simulink model "Lab6_1"  (R2025a)
settings: Solver=FixedStepDiscrete  StartTime=0.0  StopTime=A.len*16 + 52  FixedStep=1  RelTol=1e-3
PostLoadFcn:
  | A = DEScfg_axi('$0102040810204080', 'This is a default input - make it your own!', 'encrypt')
undefined symbols (not defined in the file): AXI4, Lite, xc7z020clg484
libraries: hdlBasic x260, vmcUtilities x1
(part 2 of 2)

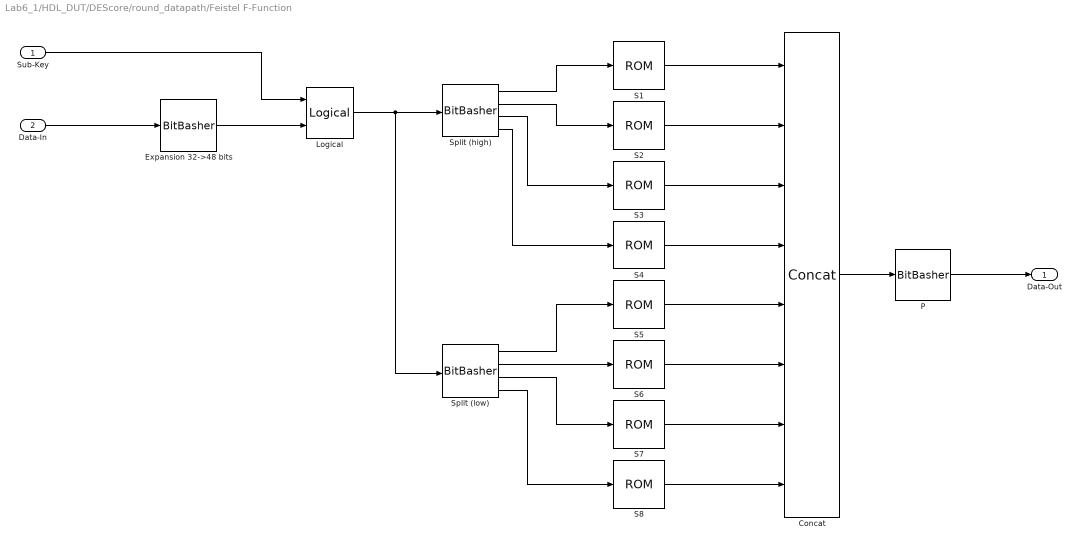
== system Lab6_1/HDL_DUT/DEScore/round_datapath/Feistel F-Function ==
  Sub-Key : Inport
  Data-In : Inport  Port=2
  Concat : hdlBasic/Concat  num_inputs=8  XmcBlockStatus=1  maskContainerNames=group1  block_type=concat  block_config=sysgen:Concat_config
  Expansion 32->48 bits : hdlBasic/BitBasher  bitexpr=x={a[0],a[31:27],a[28:23],a[24:19],a[20:15],a[16:11],a[12:7],a[8:3],a[4:0],a[31]}  display_expr=off  sr_1=x  arith_type1=Unsigned  bin_pt1=0  sr_2=y  arith_type2=Unsigned  bin_pt2=0  sr_3=z  arith_type3=Unsigned  bin_pt3=0  sr_4=t  arith_type4=Unsigned  bin_pt4=0  XmcBlockStatus=1  maskContainerNames=group1  block_type=bitbasher  block_config=sysgen:BitBasher_config
  Logical : hdlBasic/Logical  logical_function=XOR  inputs=2  en=off  latency=0  precision=Full  arith_type=Unsigned  n_bits=16  bin_pt=0  align_bp=on  overflow=[]  quantization=[]  XmcBlockStatus=1  maskContainerNames=tabcontainer1  block_type=logical  block_config=sysgen:Logical_config
  P : hdlBasic/BitBasher  bitexpr=out={a[16], a[25], a[12], a[11], a[3], a[20], a[4], a[15], a[31], a[17], a[9], a[6], a[27], a[14], a[1], a[22], a[30], a[24], a[8], a[18], a[0], a[5], a[29], a[23], a[13], a[19], a[2], a[26], a[10], a[21], a[28], a[7]}  display_expr=off  sr_1=out  arith_type1=Unsigned  bin_pt1=0  sr_2=2  arith_type2=Unsigned  bin_pt2=0  sr_3=3  arith_type3=Unsigned  bin_pt3=0  sr_4=4  arith_type4=Unsigned  bin_pt4=0  XmcBlockStatus=1  maskContainerNames=group1  block_type=bitbasher  block_config=sysgen:BitBasher_config
  S1 : hdlBasic/ROM  depth=64  initVector=[14 0 4 15 13 7 1 4 2 14 15 2 11 13 8 1 3 10 10 6 6 12 12 11 5 9 9 5 0 3 7 8 4 15 1 12 14 8 8 2 13 4 6 9 2 1 11 7 15 5 12 11 9 3 7 14 3 10 10 0 5 6 0 13]  distributed_mem=Distributed memory  rst=off  init_reg=0  en=off  latency=0  gui_display_data_type=Fixed-point  arith_type=Unsigned  n_bits=4  bin_pt=0  preci_type=Single  exp_width=8  frac_width=24  optimize=Area  use_rpm=on  simulation_type=fast_sim  XmcBlockStatus=1  maskContainerNames=tabcontainer1  block_type=sprom  block_config=sysgen:SPROM_config
  S2 : hdlBasic/ROM  depth=64  initVector=[15 3 1 13 8 4 14 7 6 15 11 2 3 8 4 14 9 12 7 0 2 1 13 10 12 6 0 9 5 11 10 5 0 13 14 8 7 10 11 1 10 3 4 15 13 4 1 2 5 11 8 6 12 7 6 12 9 0 3 5 2 14 15 9]  distributed_mem=Distributed memory  rst=off  init_reg=0  en=off  latency=0  gui_display_data_type=Fixed-point  arith_type=Unsigned  n_bits=4  bin_pt=0  preci_type=Single  exp_width=8  frac_width=24  optimize=Area  use_rpm=on  simulation_type=fast_sim  XmcBlockStatus=1  maskContainerNames=tabcontainer1  block_type=sprom  block_config=sysgen:SPROM_config
  S3 : hdlBasic/ROM  depth=64  initVector=[10 13 0 7 9 0 14 9 6 3 3 4 15 6 5 10 1 2 13 8 12 5 7 14 11 12 4 11 2 15 8 1 13 1 6 10 4 13 9 0 8 6 15 9 3 8 0 7 11 4 1 15 2 14 12 3 5 11 10 5 14 2 7 12]  distributed_mem=Distributed memory  rst=off  init_reg=0  en=off  latency=0  gui_display_data_type=Fixed-point  arith_type=Unsigned  n_bits=4  bin_pt=0  preci_type=Single  exp_width=8  frac_width=24  optimize=Area  use_rpm=on  simulation_type=fast_sim  XmcBlockStatus=1  maskContainerNames=tabcontainer1  block_type=sprom  block_config=sysgen:SPROM_config
  S4 : hdlBasic/ROM  depth=64  initVector=[7 13 13 8 14 11 3 5 0 6 6 15 9 0 10 3 1 4 2 7 8 2 5 12 11 1 12 10 4 14 15 9 10 3 6 15 9 0 0 6 12 10 11 1 7 13 13 8 15 9 1 4 3 5 14 11 5 12 2 7 8 2 4 14]  distributed_mem=Distributed memory  rst=off  init_reg=0  en=off  latency=0  gui_display_data_type=Fixed-point  arith_type=Unsigned  n_bits=4  bin_pt=0  preci_type=Single  exp_width=8  frac_width=24  optimize=Area  use_rpm=on  simulation_type=fast_sim  XmcBlockStatus=1  maskContainerNames=tabcontainer1  block_type=sprom  block_config=sysgen:SPROM_config
  S5 : hdlBasic/ROM  depth=64  initVector=[2 14 12 11 4 2 1 12 7 4 10 7 11 13 6 1 8 5 5 0 3 15 15 10 13 3 0 9 14 8 9 6 4 11 2 8 1 12 11 7 10 1 13 14 7 2 8 13 15 6 9 15 12 0 5 9 6 10 3 4 0 5 14 3]  distributed_mem=Distributed memory  rst=off  init_reg=0  en=off  latency=0  gui_display_data_type=Fixed-point  arith_type=Unsigned  n_bits=4  bin_pt=0  preci_type=Single  exp_width=8  frac_width=24  optimize=Area  use_rpm=on  simulation_type=fast_sim  XmcBlockStatus=1  maskContainerNames=tabcontainer1  block_type=sprom  block_config=sysgen:SPROM_config
  S6 : hdlBasic/ROM  depth=64  initVector=[12 10 1 15 10 4 15 2 9 7 2 12 6 9 8 5 0 6 13 1 3 13 4 14 14 0 7 11 5 3 11 8 9 4 14 3 15 2 5 12 2 9 8 5 12 15 3 10 7 11 0 14 4 1 10 7 1 6 13 0 11 8 6 13]  distributed_mem=Distributed memory  rst=off  init_reg=0  en=off  latency=0  gui_display_data_type=Fixed-point  arith_type=Unsigned  n_bits=4  bin_pt=0  preci_type=Single  exp_width=8  frac_width=24  optimize=Area  use_rpm=on  simulation_type=fast_sim  XmcBlockStatus=1  maskContainerNames=tabcontainer1  block_type=sprom  block_config=sysgen:SPROM_config
  S7 : hdlBasic/ROM  depth=64  initVector=[4 13 11 0 2 11 14 7 15 4 0 9 8 1 13 10 3 14 12 3 9 5 7 12 5 2 10 15 6 8 1 6 1 6 4 11 11 13 13 8 12 1 3 4 7 10 14 7 10 9 15 5 6 0 8 15 0 14 5 2 9 3 2 12]  distributed_mem=Distributed memory  rst=off  init_reg=0  en=off  latency=0  gui_display_data_type=Fixed-point  arith_type=Unsigned  n_bits=4  bin_pt=0  preci_type=Single  exp_width=8  frac_width=24  optimize=Area  use_rpm=on  simulation_type=fast_sim  XmcBlockStatus=1  maskContainerNames=tabcontainer1  block_type=sprom  block_config=sysgen:SPROM_config
  S8 : hdlBasic/ROM  depth=64  initVector=[13 1 2 15 8 13 4 8 6 10 15 3 11 7 1 4 10 12 9 5 3 6 14 11 5 0 0 14 12 9 7 2 7 2 11 1 4 14 1 7 9 4 12 10 14 8 2 13 0 15 6 12 10 9 13 0 15 3 3 5 5 6 8 11]  distributed_mem=Distributed memory  rst=off  init_reg=0  en=off  latency=0  gui_display_data_type=Fixed-point  arith_type=Unsigned  n_bits=4  bin_pt=0  preci_type=Single  exp_width=8  frac_width=24  optimize=Area  use_rpm=on  simulation_type=fast_sim  XmcBlockStatus=1  maskContainerNames=tabcontainer1  block_type=sprom  block_config=sysgen:SPROM_config
  Split (high) : hdlBasic/BitBasher  bitexpr=|  display_expr=off  sr_1=a  arith_type1=Unsigned  bin_pt1=0  sr_2=b  arith_type2=Unsigned  bin_pt2=0  sr_3=c  arith_type3=Unsigned  bin_pt3=0  sr_4=d  arith_type4=Unsigned  bin_pt4=0  XmcBlockStatus=1  maskContainerNames=group1  block_type=bitbasher  block_config=sysgen:BitBasher_config
      | a={x[47:42]}
      | b={x[41:36]}
      | c={x[35:30]}
      | d={x[29:24]}
  Split (low) : hdlBasic/BitBasher  bitexpr=|  display_expr=off  sr_1=a  arith_type1=Unsigned  bin_pt1=0  sr_2=b  arith_type2=Unsigned  bin_pt2=0  sr_3=c  arith_type3=Unsigned  bin_pt3=0  sr_4=d  arith_type4=Unsigned  bin_pt4=0  XmcBlockStatus=1  maskContainerNames=group1  block_type=bitbasher  block_config=sysgen:BitBasher_config
      | a={x[23:18]}
      | b={x[17:12]}
      | c={x[11:6]}
      | d={x[5:0]}
  Data-Out : Outport
  wires:
  Split (low)/2 -> S6/1
  Split (low)/3 -> S7/1
  Concat/1 -> P/1
  S4/1 -> Concat/4
  Split (low)/1 -> S5/1
  Split (high)/3 -> S3/1
  S6/1 -> Concat/6
  Split (high)/4 -> S4/1
  S8/1 -> Concat/8
  Data-In/1 -> Expansion 32->48 bits/1
  S1/1 -> Concat/1
  Logical/1 -> Split (low)/1, Split (high)/1
  Sub-Key/1 -> Logical/1
  Expansion 32->48 bits/1 -> Logical/2
  Split (low)/4 -> S8/1
  Split (high)/1 -> S1/1
  Split (high)/2 -> S2/1
  S7/1 -> Concat/7
  S5/1 -> Concat/5
  S2/1 -> Concat/2
  S3/1 -> Concat/3
  P/1 -> Data-Out/1

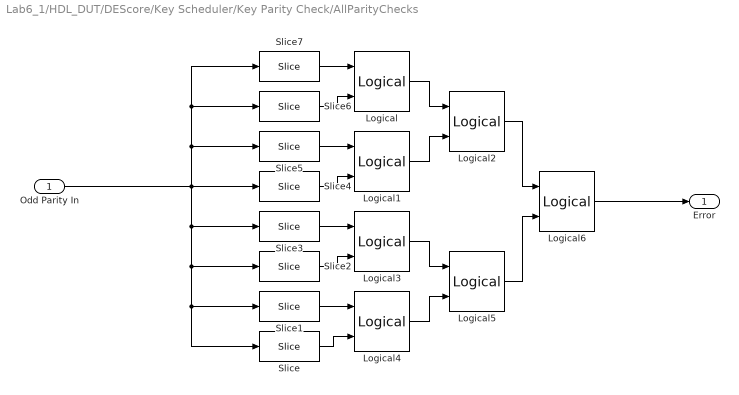
== system Lab6_1/HDL_DUT/DEScore/Key Scheduler/Key Parity Check/AllParityChecks ==
  Odd Parity In : Inport
  Logical{,1..5} (6 alike) : hdlBasic/Logical  logical_function=AND  inputs=2  en=off  latency=0  precision=Full  arith_type=Unsigned  n_bits=16  bin_pt=0  align_bp=on  overflow=[]  quantization=[]  XmcBlockStatus=1  maskContainerNames=tabcontainer1  block_type=logical  block_config=sysgen:Logical_config
  Logical6 : hdlBasic/Logical  logical_function=NAND  inputs=2  en=off  latency=0  precision=Full  arith_type=Unsigned  n_bits=16  bin_pt=0  align_bp=on  overflow=[]  quantization=[]  XmcBlockStatus=1  maskContainerNames=tabcontainer1  block_type=logical  block_config=sysgen:Logical_config
  Slice : hdlBasic/Slice  nbits=1  boolean_output=on  mode=Upper Bit Location + Width  bit1=0  base1=LSB of Input  bit0=0  base0=LSB of Input  XmcBlockStatus=1  maskContainerNames=group1  block_type=slice  block_config=sysgen:Slice_config
  Slice1 : hdlBasic/Slice  nbits=1  boolean_output=on  mode=Upper Bit Location + Width  bit1=1  base1=LSB of Input  bit0=0  base0=LSB of Input  XmcBlockStatus=1  maskContainerNames=group1  block_type=slice  block_config=sysgen:Slice_config
  Slice2 : hdlBasic/Slice  nbits=1  boolean_output=on  mode=Upper Bit Location + Width  bit1=2  base1=LSB of Input  bit0=0  base0=LSB of Input  XmcBlockStatus=1  maskContainerNames=group1  block_type=slice  block_config=sysgen:Slice_config
  Slice3 : hdlBasic/Slice  nbits=1  boolean_output=on  mode=Upper Bit Location + Width  bit1=3  base1=LSB of Input  bit0=0  base0=LSB of Input  XmcBlockStatus=1  maskContainerNames=group1  block_type=slice  block_config=sysgen:Slice_config
  Slice4 : hdlBasic/Slice  nbits=1  boolean_output=on  mode=Upper Bit Location + Width  bit1=4  base1=LSB of Input  bit0=0  base0=LSB of Input  XmcBlockStatus=1  maskContainerNames=group1  block_type=slice  block_config=sysgen:Slice_config
  Slice5 : hdlBasic/Slice  nbits=1  boolean_output=on  mode=Upper Bit Location + Width  bit1=5  base1=LSB of Input  bit0=0  base0=LSB of Input  XmcBlockStatus=1  maskContainerNames=group1  block_type=slice  block_config=sysgen:Slice_config
  Slice6 : hdlBasic/Slice  nbits=1  boolean_output=on  mode=Upper Bit Location + Width  bit1=6  base1=LSB of Input  bit0=0  base0=LSB of Input  XmcBlockStatus=1  maskContainerNames=group1  block_type=slice  block_config=sysgen:Slice_config
  Slice7 : hdlBasic/Slice  nbits=1  boolean_output=on  mode=Upper Bit Location + Width  bit1=7  base1=LSB of Input  bit0=0  base0=LSB of Input  XmcBlockStatus=1  maskContainerNames=group1  block_type=slice  block_config=sysgen:Slice_config
  Error : Outport
  wires:
  Logical/1 -> Logical2/1
  Slice3/1 -> Logical3/1
  Slice1/1 -> Logical4/1
  Logical2/1 -> Logical6/1
  Logical1/1 -> Logical2/2
  Slice/1 -> Logical4/2
  Slice4/1 -> Logical1/2
  Slice5/1 -> Logical1/1
  Logical4/1 -> Logical5/2
  Logical3/1 -> Logical5/1
  Slice7/1 -> Logical/1
  Slice6/1 -> Logical/2
  Slice2/1 -> Logical3/2
  Logical5/1 -> Logical6/2
  Odd Parity In/1 -> Slice7/1, Slice6/1, Slice5/1, Slice/1, Slice1/1, Slice2/1, Slice3/1, Slice4/1
  Logical6/1 -> Error/1

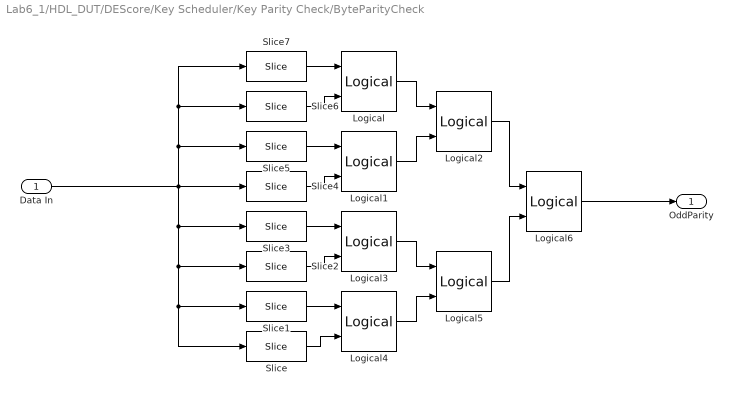
== system Lab6_1/HDL_DUT/DEScore/Key Scheduler/Key Parity Check/ByteParityCheck ==
  Data In : Inport
  Logical{,1..6} (7 alike) : hdlBasic/Logical  logical_function=XOR  inputs=2  en=off  latency=0  precision=Full  arith_type=Unsigned  n_bits=16  bin_pt=0  align_bp=on  overflow=[]  quantization=[]  XmcBlockStatus=1  maskContainerNames=tabcontainer1  block_type=logical  block_config=sysgen:Logical_config
  Slice : hdlBasic/Slice  nbits=1  boolean_output=on  mode=Upper Bit Location + Width  bit1=0  base1=LSB of Input  bit0=0  base0=LSB of Input  XmcBlockStatus=1  maskContainerNames=group1  block_type=slice  block_config=sysgen:Slice_config
  Slice1 : hdlBasic/Slice  nbits=1  boolean_output=on  mode=Upper Bit Location + Width  bit1=1  base1=LSB of Input  bit0=0  base0=LSB of Input  XmcBlockStatus=1  maskContainerNames=group1  block_type=slice  block_config=sysgen:Slice_config
  Slice2 : hdlBasic/Slice  nbits=1  boolean_output=on  mode=Upper Bit Location + Width  bit1=2  base1=LSB of Input  bit0=0  base0=LSB of Input  XmcBlockStatus=1  maskContainerNames=group1  block_type=slice  block_config=sysgen:Slice_config
  Slice3 : hdlBasic/Slice  nbits=1  boolean_output=on  mode=Upper Bit Location + Width  bit1=3  base1=LSB of Input  bit0=0  base0=LSB of Input  XmcBlockStatus=1  maskContainerNames=group1  block_type=slice  block_config=sysgen:Slice_config
  Slice4 : hdlBasic/Slice  nbits=1  boolean_output=on  mode=Upper Bit Location + Width  bit1=4  base1=LSB of Input  bit0=0  base0=LSB of Input  XmcBlockStatus=1  maskContainerNames=group1  block_type=slice  block_config=sysgen:Slice_config
  Slice5 : hdlBasic/Slice  nbits=1  boolean_output=on  mode=Upper Bit Location + Width  bit1=5  base1=LSB of Input  bit0=0  base0=LSB of Input  XmcBlockStatus=1  maskContainerNames=group1  block_type=slice  block_config=sysgen:Slice_config
  Slice6 : hdlBasic/Slice  nbits=1  boolean_output=on  mode=Upper Bit Location + Width  bit1=6  base1=LSB of Input  bit0=0  base0=LSB of Input  XmcBlockStatus=1  maskContainerNames=group1  block_type=slice  block_config=sysgen:Slice_config
  Slice7 : hdlBasic/Slice  nbits=1  boolean_output=on  mode=Upper Bit Location + Width  bit1=7  base1=LSB of Input  bit0=0  base0=LSB of Input  XmcBlockStatus=1  maskContainerNames=group1  block_type=slice  block_config=sysgen:Slice_config
  OddParity : Outport
  wires:
  Logical/1 -> Logical2/1
  Slice3/1 -> Logical3/1
  Slice1/1 -> Logical4/1
  Logical2/1 -> Logical6/1
  Logical1/1 -> Logical2/2
  Slice/1 -> Logical4/2
  Slice4/1 -> Logical1/2
  Slice5/1 -> Logical1/1
  Logical4/1 -> Logical5/2
  Logical3/1 -> Logical5/1
  Slice7/1 -> Logical/1
  Slice6/1 -> Logical/2
  Slice2/1 -> Logical3/2
  Logical5/1 -> Logical6/2
  Data In/1 -> Slice7/1, Slice6/1, Slice5/1, Slice/1, Slice1/1, Slice2/1, Slice3/1, Slice4/1
  Logical6/1 -> OddParity/1

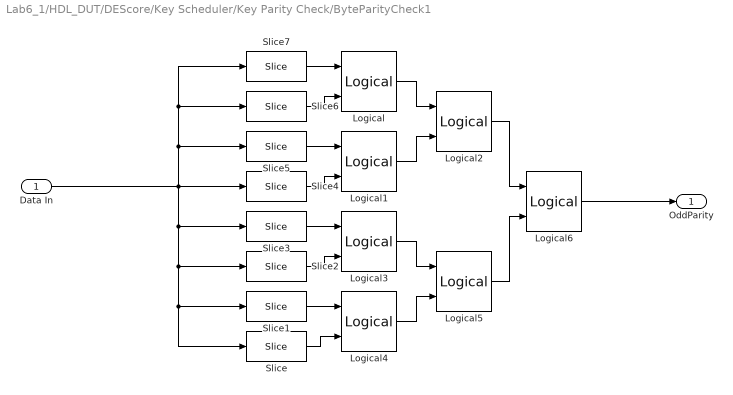
== system Lab6_1/HDL_DUT/DEScore/Key Scheduler/Key Parity Check/ByteParityCheck1 ==
  Data In : Inport
  Logical{,1..6} (7 alike) : hdlBasic/Logical  logical_function=XOR  inputs=2  en=off  latency=0  precision=Full  arith_type=Unsigned  n_bits=16  bin_pt=0  align_bp=on  overflow=[]  quantization=[]  XmcBlockStatus=1  maskContainerNames=tabcontainer1  block_type=logical  block_config=sysgen:Logical_config
  Slice : hdlBasic/Slice  nbits=1  boolean_output=on  mode=Upper Bit Location + Width  bit1=0  base1=LSB of Input  bit0=0  base0=LSB of Input  XmcBlockStatus=1  maskContainerNames=group1  block_type=slice  block_config=sysgen:Slice_config
  Slice1 : hdlBasic/Slice  nbits=1  boolean_output=on  mode=Upper Bit Location + Width  bit1=1  base1=LSB of Input  bit0=0  base0=LSB of Input  XmcBlockStatus=1  maskContainerNames=group1  block_type=slice  block_config=sysgen:Slice_config
  Slice2 : hdlBasic/Slice  nbits=1  boolean_output=on  mode=Upper Bit Location + Width  bit1=2  base1=LSB of Input  bit0=0  base0=LSB of Input  XmcBlockStatus=1  maskContainerNames=group1  block_type=slice  block_config=sysgen:Slice_config
  Slice3 : hdlBasic/Slice  nbits=1  boolean_output=on  mode=Upper Bit Location + Width  bit1=3  base1=LSB of Input  bit0=0  base0=LSB of Input  XmcBlockStatus=1  maskContainerNames=group1  block_type=slice  block_config=sysgen:Slice_config
  Slice4 : hdlBasic/Slice  nbits=1  boolean_output=on  mode=Upper Bit Location + Width  bit1=4  base1=LSB of Input  bit0=0  base0=LSB of Input  XmcBlockStatus=1  maskContainerNames=group1  block_type=slice  block_config=sysgen:Slice_config
  Slice5 : hdlBasic/Slice  nbits=1  boolean_output=on  mode=Upper Bit Location + Width  bit1=5  base1=LSB of Input  bit0=0  base0=LSB of Input  XmcBlockStatus=1  maskContainerNames=group1  block_type=slice  block_config=sysgen:Slice_config
  Slice6 : hdlBasic/Slice  nbits=1  boolean_output=on  mode=Upper Bit Location + Width  bit1=6  base1=LSB of Input  bit0=0  base0=LSB of Input  XmcBlockStatus=1  maskContainerNames=group1  block_type=slice  block_config=sysgen:Slice_config
  Slice7 : hdlBasic/Slice  nbits=1  boolean_output=on  mode=Upper Bit Location + Width  bit1=7  base1=LSB of Input  bit0=0  base0=LSB of Input  XmcBlockStatus=1  maskContainerNames=group1  block_type=slice  block_config=sysgen:Slice_config
  OddParity : Outport
  wires:
  Logical/1 -> Logical2/1
  Slice3/1 -> Logical3/1
  Slice1/1 -> Logical4/1
  Logical2/1 -> Logical6/1
  Logical1/1 -> Logical2/2
  Slice/1 -> Logical4/2
  Slice4/1 -> Logical1/2
  Slice5/1 -> Logical1/1
  Logical4/1 -> Logical5/2
  Logical3/1 -> Logical5/1
  Slice7/1 -> Logical/1
  Slice6/1 -> Logical/2
  Slice2/1 -> Logical3/2
  Logical5/1 -> Logical6/2
  Data In/1 -> Slice7/1, Slice6/1, Slice5/1, Slice/1, Slice1/1, Slice2/1, Slice3/1, Slice4/1
  Logical6/1 -> OddParity/1

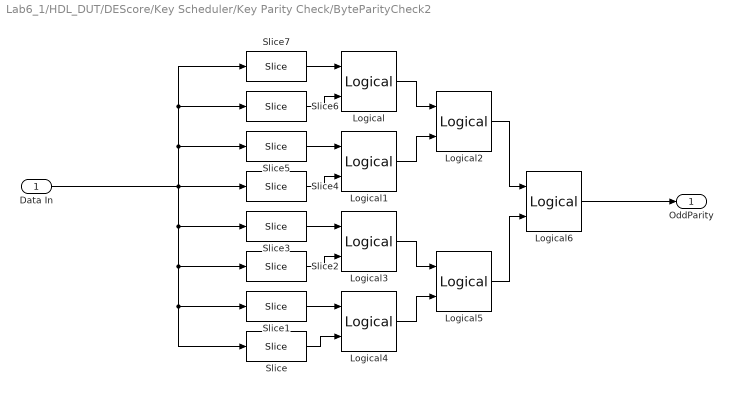
== system Lab6_1/HDL_DUT/DEScore/Key Scheduler/Key Parity Check/ByteParityCheck2 ==
  Data In : Inport
  Logical{,1..6} (7 alike) : hdlBasic/Logical  logical_function=XOR  inputs=2  en=off  latency=0  precision=Full  arith_type=Unsigned  n_bits=16  bin_pt=0  align_bp=on  overflow=[]  quantization=[]  XmcBlockStatus=1  maskContainerNames=tabcontainer1  block_type=logical  block_config=sysgen:Logical_config
  Slice : hdlBasic/Slice  nbits=1  boolean_output=on  mode=Upper Bit Location + Width  bit1=0  base1=LSB of Input  bit0=0  base0=LSB of Input  XmcBlockStatus=1  maskContainerNames=group1  block_type=slice  block_config=sysgen:Slice_config
  Slice1 : hdlBasic/Slice  nbits=1  boolean_output=on  mode=Upper Bit Location + Width  bit1=1  base1=LSB of Input  bit0=0  base0=LSB of Input  XmcBlockStatus=1  maskContainerNames=group1  block_type=slice  block_config=sysgen:Slice_config
  Slice2 : hdlBasic/Slice  nbits=1  boolean_output=on  mode=Upper Bit Location + Width  bit1=2  base1=LSB of Input  bit0=0  base0=LSB of Input  XmcBlockStatus=1  maskContainerNames=group1  block_type=slice  block_config=sysgen:Slice_config
  Slice3 : hdlBasic/Slice  nbits=1  boolean_output=on  mode=Upper Bit Location + Width  bit1=3  base1=LSB of Input  bit0=0  base0=LSB of Input  XmcBlockStatus=1  maskContainerNames=group1  block_type=slice  block_config=sysgen:Slice_config
  Slice4 : hdlBasic/Slice  nbits=1  boolean_output=on  mode=Upper Bit Location + Width  bit1=4  base1=LSB of Input  bit0=0  base0=LSB of Input  XmcBlockStatus=1  maskContainerNames=group1  block_type=slice  block_config=sysgen:Slice_config
  Slice5 : hdlBasic/Slice  nbits=1  boolean_output=on  mode=Upper Bit Location + Width  bit1=5  base1=LSB of Input  bit0=0  base0=LSB of Input  XmcBlockStatus=1  maskContainerNames=group1  block_type=slice  block_config=sysgen:Slice_config
  Slice6 : hdlBasic/Slice  nbits=1  boolean_output=on  mode=Upper Bit Location + Width  bit1=6  base1=LSB of Input  bit0=0  base0=LSB of Input  XmcBlockStatus=1  maskContainerNames=group1  block_type=slice  block_config=sysgen:Slice_config
  Slice7 : hdlBasic/Slice  nbits=1  boolean_output=on  mode=Upper Bit Location + Width  bit1=7  base1=LSB of Input  bit0=0  base0=LSB of Input  XmcBlockStatus=1  maskContainerNames=group1  block_type=slice  block_config=sysgen:Slice_config
  OddParity : Outport
  wires:
  Logical/1 -> Logical2/1
  Slice3/1 -> Logical3/1
  Slice1/1 -> Logical4/1
  Logical2/1 -> Logical6/1
  Logical1/1 -> Logical2/2
  Slice/1 -> Logical4/2
  Slice4/1 -> Logical1/2
  Slice5/1 -> Logical1/1
  Logical4/1 -> Logical5/2
  Logical3/1 -> Logical5/1
  Slice7/1 -> Logical/1
  Slice6/1 -> Logical/2
  Slice2/1 -> Logical3/2
  Logical5/1 -> Logical6/2
  Data In/1 -> Slice7/1, Slice6/1, Slice5/1, Slice/1, Slice1/1, Slice2/1, Slice3/1, Slice4/1
  Logical6/1 -> OddParity/1

== system Lab6_1/HDL_DUT/DEScore/Key Scheduler/Key Parity Check/ByteParityCheck3 ==
  Data In : Inport
  Logical{,1..6} (7 alike) : hdlBasic/Logical  logical_function=XOR  inputs=2  en=off  latency=0  precision=Full  arith_type=Unsigned  n_bits=16  bin_pt=0  align_bp=on  overflow=[]  quantization=[]  XmcBlockStatus=1  maskContainerNames=tabcontainer1  block_type=logical  block_config=sysgen:Logical_config
  Slice : hdlBasic/Slice  nbits=1  boolean_output=on  mode=Upper Bit Location + Width  bit1=0  base1=LSB of Input  bit0=0  base0=LSB of Input  XmcBlockStatus=1  maskContainerNames=group1  block_type=slice  block_config=sysgen:Slice_config
  Slice1 : hdlBasic/Slice  nbits=1  boolean_output=on  mode=Upper Bit Location + Width  bit1=1  base1=LSB of Input  bit0=0  base0=LSB of Input  XmcBlockStatus=1  maskContainerNames=group1  block_type=slice  block_config=sysgen:Slice_config
  Slice2 : hdlBasic/Slice  nbits=1  boolean_output=on  mode=Upper Bit Location + Width  bit1=2  base1=LSB of Input  bit0=0  base0=LSB of Input  XmcBlockStatus=1  maskContainerNames=group1  block_type=slice  block_config=sysgen:Slice_config
  Slice3 : hdlBasic/Slice  nbits=1  boolean_output=on  mode=Upper Bit Location + Width  bit1=3  base1=LSB of Input  bit0=0  base0=LSB of Input  XmcBlockStatus=1  maskContainerNames=group1  block_type=slice  block_config=sysgen:Slice_config
  Slice4 : hdlBasic/Slice  nbits=1  boolean_output=on  mode=Upper Bit Location + Width  bit1=4  base1=LSB of Input  bit0=0  base0=LSB of Input  XmcBlockStatus=1  maskContainerNames=group1  block_type=slice  block_config=sysgen:Slice_config
  Slice5 : hdlBasic/Slice  nbits=1  boolean_output=on  mode=Upper Bit Location + Width  bit1=5  base1=LSB of Input  bit0=0  base0=LSB of Input  XmcBlockStatus=1  maskContainerNames=group1  block_type=slice  block_config=sysgen:Slice_config
  Slice6 : hdlBasic/Slice  nbits=1  boolean_output=on  mode=Upper Bit Location + Width  bit1=6  base1=LSB of Input  bit0=0  base0=LSB of Input  XmcBlockStatus=1  maskContainerNames=group1  block_type=slice  block_config=sysgen:Slice_config
  Slice7 : hdlBasic/Slice  nbits=1  boolean_output=on  mode=Upper Bit Location + Width  bit1=7  base1=LSB of Input  bit0=0  base0=LSB of Input  XmcBlockStatus=1  maskContainerNames=group1  block_type=slice  block_config=sysgen:Slice_config
  OddParity : Outport
  wires:
  Logical/1 -> Logical2/1
  Slice3/1 -> Logical3/1
  Slice1/1 -> Logical4/1
  Logical2/1 -> Logical6/1
  Logical1/1 -> Logical2/2
  Slice/1 -> Logical4/2
  Slice4/1 -> Logical1/2
  Slice5/1 -> Logical1/1
  Logical4/1 -> Logical5/2
  Logical3/1 -> Logical5/1
  Slice7/1 -> Logical/1
  Slice6/1 -> Logical/2
  Slice2/1 -> Logical3/2
  Logical5/1 -> Logical6/2
  Data In/1 -> Slice7/1, Slice6/1, Slice5/1, Slice/1, Slice1/1, Slice2/1, Slice3/1, Slice4/1
  Logical6/1 -> OddParity/1

== system Lab6_1/HDL_DUT/DEScore/Key Scheduler/Key Parity Check/ByteParityCheck4 ==
  Data In : Inport
  Logical{,1..6} (7 alike) : hdlBasic/Logical  logical_function=XOR  inputs=2  en=off  latency=0  precision=Full  arith_type=Unsigned  n_bits=16  bin_pt=0  align_bp=on  overflow=[]  quantization=[]  XmcBlockStatus=1  maskContainerNames=tabcontainer1  block_type=logical  block_config=sysgen:Logical_config
  Slice : hdlBasic/Slice  nbits=1  boolean_output=on  mode=Upper Bit Location + Width  bit1=0  base1=LSB of Input  bit0=0  base0=LSB of Input  XmcBlockStatus=1  maskContainerNames=group1  block_type=slice  block_config=sysgen:Slice_config
  Slice1 : hdlBasic/Slice  nbits=1  boolean_output=on  mode=Upper Bit Location + Width  bit1=1  base1=LSB of Input  bit0=0  base0=LSB of Input  XmcBlockStatus=1  maskContainerNames=group1  block_type=slice  block_config=sysgen:Slice_config
  Slice2 : hdlBasic/Slice  nbits=1  boolean_output=on  mode=Upper Bit Location + Width  bit1=2  base1=LSB of Input  bit0=0  base0=LSB of Input  XmcBlockStatus=1  maskContainerNames=group1  block_type=slice  block_config=sysgen:Slice_config
  Slice3 : hdlBasic/Slice  nbits=1  boolean_output=on  mode=Upper Bit Location + Width  bit1=3  base1=LSB of Input  bit0=0  base0=LSB of Input  XmcBlockStatus=1  maskContainerNames=group1  block_type=slice  block_config=sysgen:Slice_config
  Slice4 : hdlBasic/Slice  nbits=1  boolean_output=on  mode=Upper Bit Location + Width  bit1=4  base1=LSB of Input  bit0=0  base0=LSB of Input  XmcBlockStatus=1  maskContainerNames=group1  block_type=slice  block_config=sysgen:Slice_config
  Slice5 : hdlBasic/Slice  nbits=1  boolean_output=on  mode=Upper Bit Location + Width  bit1=5  base1=LSB of Input  bit0=0  base0=LSB of Input  XmcBlockStatus=1  maskContainerNames=group1  block_type=slice  block_config=sysgen:Slice_config
  Slice6 : hdlBasic/Slice  nbits=1  boolean_output=on  mode=Upper Bit Location + Width  bit1=6  base1=LSB of Input  bit0=0  base0=LSB of Input  XmcBlockStatus=1  maskContainerNames=group1  block_type=slice  block_config=sysgen:Slice_config
  Slice7 : hdlBasic/Slice  nbits=1  boolean_output=on  mode=Upper Bit Location + Width  bit1=7  base1=LSB of Input  bit0=0  base0=LSB of Input  XmcBlockStatus=1  maskContainerNames=group1  block_type=slice  block_config=sysgen:Slice_config
  OddParity : Outport
  wires:
  Logical/1 -> Logical2/1
  Slice3/1 -> Logical3/1
  Slice1/1 -> Logical4/1
  Logical2/1 -> Logical6/1
  Logical1/1 -> Logical2/2
  Slice/1 -> Logical4/2
  Slice4/1 -> Logical1/2
  Slice5/1 -> Logical1/1
  Logical4/1 -> Logical5/2
  Logical3/1 -> Logical5/1
  Slice7/1 -> Logical/1
  Slice6/1 -> Logical/2
  Slice2/1 -> Logical3/2
  Logical5/1 -> Logical6/2
  Data In/1 -> Slice7/1, Slice6/1, Slice5/1, Slice/1, Slice1/1, Slice2/1, Slice3/1, Slice4/1
  Logical6/1 -> OddParity/1

== system Lab6_1/HDL_DUT/DEScore/Key Scheduler/Key Parity Check/ByteParityCheck5 ==
  Data In : Inport
  Logical{,1..6} (7 alike) : hdlBasic/Logical  logical_function=XOR  inputs=2  en=off  latency=0  precision=Full  arith_type=Unsigned  n_bits=16  bin_pt=0  align_bp=on  overflow=[]  quantization=[]  XmcBlockStatus=1  maskContainerNames=tabcontainer1  block_type=logical  block_config=sysgen:Logical_config
  Slice : hdlBasic/Slice  nbits=1  boolean_output=on  mode=Upper Bit Location + Width  bit1=0  base1=LSB of Input  bit0=0  base0=LSB of Input  XmcBlockStatus=1  maskContainerNames=group1  block_type=slice  block_config=sysgen:Slice_config
  Slice1 : hdlBasic/Slice  nbits=1  boolean_output=on  mode=Upper Bit Location + Width  bit1=1  base1=LSB of Input  bit0=0  base0=LSB of Input  XmcBlockStatus=1  maskContainerNames=group1  block_type=slice  block_config=sysgen:Slice_config
  Slice2 : hdlBasic/Slice  nbits=1  boolean_output=on  mode=Upper Bit Location + Width  bit1=2  base1=LSB of Input  bit0=0  base0=LSB of Input  XmcBlockStatus=1  maskContainerNames=group1  block_type=slice  block_config=sysgen:Slice_config
  Slice3 : hdlBasic/Slice  nbits=1  boolean_output=on  mode=Upper Bit Location + Width  bit1=3  base1=LSB of Input  bit0=0  base0=LSB of Input  XmcBlockStatus=1  maskContainerNames=group1  block_type=slice  block_config=sysgen:Slice_config
  Slice4 : hdlBasic/Slice  nbits=1  boolean_output=on  mode=Upper Bit Location + Width  bit1=4  base1=LSB of Input  bit0=0  base0=LSB of Input  XmcBlockStatus=1  maskContainerNames=group1  block_type=slice  block_config=sysgen:Slice_config
  Slice5 : hdlBasic/Slice  nbits=1  boolean_output=on  mode=Upper Bit Location + Width  bit1=5  base1=LSB of Input  bit0=0  base0=LSB of Input  XmcBlockStatus=1  maskContainerNames=group1  block_type=slice  block_config=sysgen:Slice_config
  Slice6 : hdlBasic/Slice  nbits=1  boolean_output=on  mode=Upper Bit Location + Width  bit1=6  base1=LSB of Input  bit0=0  base0=LSB of Input  XmcBlockStatus=1  maskContainerNames=group1  block_type=slice  block_config=sysgen:Slice_config
  Slice7 : hdlBasic/Slice  nbits=1  boolean_output=on  mode=Upper Bit Location + Width  bit1=7  base1=LSB of Input  bit0=0  base0=LSB of Input  XmcBlockStatus=1  maskContainerNames=group1  block_type=slice  block_config=sysgen:Slice_config
  OddParity : Outport
  wires:
  Logical/1 -> Logical2/1
  Slice3/1 -> Logical3/1
  Slice1/1 -> Logical4/1
  Logical2/1 -> Logical6/1
  Logical1/1 -> Logical2/2
  Slice/1 -> Logical4/2
  Slice4/1 -> Logical1/2
  Slice5/1 -> Logical1/1
  Logical4/1 -> Logical5/2
  Logical3/1 -> Logical5/1
  Slice7/1 -> Logical/1
  Slice6/1 -> Logical/2
  Slice2/1 -> Logical3/2
  Logical5/1 -> Logical6/2
  Data In/1 -> Slice7/1, Slice6/1, Slice5/1, Slice/1, Slice1/1, Slice2/1, Slice3/1, Slice4/1
  Logical6/1 -> OddParity/1

== system Lab6_1/HDL_DUT/DEScore/Key Scheduler/Key Parity Check/ByteParityCheck6 ==
  Data In : Inport
  Logical{,1..6} (7 alike) : hdlBasic/Logical  logical_function=XOR  inputs=2  en=off  latency=0  precision=Full  arith_type=Unsigned  n_bits=16  bin_pt=0  align_bp=on  overflow=[]  quantization=[]  XmcBlockStatus=1  maskContainerNames=tabcontainer1  block_type=logical  block_config=sysgen:Logical_config
  Slice : hdlBasic/Slice  nbits=1  boolean_output=on  mode=Upper Bit Location + Width  bit1=0  base1=LSB of Input  bit0=0  base0=LSB of Input  XmcBlockStatus=1  maskContainerNames=group1  block_type=slice  block_config=sysgen:Slice_config
  Slice1 : hdlBasic/Slice  nbits=1  boolean_output=on  mode=Upper Bit Location + Width  bit1=1  base1=LSB of Input  bit0=0  base0=LSB of Input  XmcBlockStatus=1  maskContainerNames=group1  block_type=slice  block_config=sysgen:Slice_config
  Slice2 : hdlBasic/Slice  nbits=1  boolean_output=on  mode=Upper Bit Location + Width  bit1=2  base1=LSB of Input  bit0=0  base0=LSB of Input  XmcBlockStatus=1  maskContainerNames=group1  block_type=slice  block_config=sysgen:Slice_config
  Slice3 : hdlBasic/Slice  nbits=1  boolean_output=on  mode=Upper Bit Location + Width  bit1=3  base1=LSB of Input  bit0=0  base0=LSB of Input  XmcBlockStatus=1  maskContainerNames=group1  block_type=slice  block_config=sysgen:Slice_config
  Slice4 : hdlBasic/Slice  nbits=1  boolean_output=on  mode=Upper Bit Location + Width  bit1=4  base1=LSB of Input  bit0=0  base0=LSB of Input  XmcBlockStatus=1  maskContainerNames=group1  block_type=slice  block_config=sysgen:Slice_config
  Slice5 : hdlBasic/Slice  nbits=1  boolean_output=on  mode=Upper Bit Location + Width  bit1=5  base1=LSB of Input  bit0=0  base0=LSB of Input  XmcBlockStatus=1  maskContainerNames=group1  block_type=slice  block_config=sysgen:Slice_config
  Slice6 : hdlBasic/Slice  nbits=1  boolean_output=on  mode=Upper Bit Location + Width  bit1=6  base1=LSB of Input  bit0=0  base0=LSB of Input  XmcBlockStatus=1  maskContainerNames=group1  block_type=slice  block_config=sysgen:Slice_config
  Slice7 : hdlBasic/Slice  nbits=1  boolean_output=on  mode=Upper Bit Location + Width  bit1=7  base1=LSB of Input  bit0=0  base0=LSB of Input  XmcBlockStatus=1  maskContainerNames=group1  block_type=slice  block_config=sysgen:Slice_config
  OddParity : Outport
  wires:
  Logical/1 -> Logical2/1
  Slice3/1 -> Logical3/1
  Slice1/1 -> Logical4/1
  Logical2/1 -> Logical6/1
  Logical1/1 -> Logical2/2
  Slice/1 -> Logical4/2
  Slice4/1 -> Logical1/2
  Slice5/1 -> Logical1/1
  Logical4/1 -> Logical5/2
  Logical3/1 -> Logical5/1
  Slice7/1 -> Logical/1
  Slice6/1 -> Logical/2
  Slice2/1 -> Logical3/2
  Logical5/1 -> Logical6/2
  Data In/1 -> Slice7/1, Slice6/1, Slice5/1, Slice/1, Slice1/1, Slice2/1, Slice3/1, Slice4/1
  Logical6/1 -> OddParity/1

== system Lab6_1/HDL_DUT/DEScore/Key Scheduler/Key Parity Check/ByteParityCheck7 ==
  Data In : Inport
  Logical{,1..6} (7 alike) : hdlBasic/Logical  logical_function=XOR  inputs=2  en=off  latency=0  precision=Full  arith_type=Unsigned  n_bits=16  bin_pt=0  align_bp=on  overflow=[]  quantization=[]  XmcBlockStatus=1  maskContainerNames=tabcontainer1  block_type=logical  block_config=sysgen:Logical_config
  Slice : hdlBasic/Slice  nbits=1  boolean_output=on  mode=Upper Bit Location + Width  bit1=0  base1=LSB of Input  bit0=0  base0=LSB of Input  XmcBlockStatus=1  maskContainerNames=group1  block_type=slice  block_config=sysgen:Slice_config
  Slice1 : hdlBasic/Slice  nbits=1  boolean_output=on  mode=Upper Bit Location + Width  bit1=1  base1=LSB of Input  bit0=0  base0=LSB of Input  XmcBlockStatus=1  maskContainerNames=group1  block_type=slice  block_config=sysgen:Slice_config
  Slice2 : hdlBasic/Slice  nbits=1  boolean_output=on  mode=Upper Bit Location + Width  bit1=2  base1=LSB of Input  bit0=0  base0=LSB of Input  XmcBlockStatus=1  maskContainerNames=group1  block_type=slice  block_config=sysgen:Slice_config
  Slice3 : hdlBasic/Slice  nbits=1  boolean_output=on  mode=Upper Bit Location + Width  bit1=3  base1=LSB of Input  bit0=0  base0=LSB of Input  XmcBlockStatus=1  maskContainerNames=group1  block_type=slice  block_config=sysgen:Slice_config
  Slice4 : hdlBasic/Slice  nbits=1  boolean_output=on  mode=Upper Bit Location + Width  bit1=4  base1=LSB of Input  bit0=0  base0=LSB of Input  XmcBlockStatus=1  maskContainerNames=group1  block_type=slice  block_config=sysgen:Slice_config
  Slice5 : hdlBasic/Slice  nbits=1  boolean_output=on  mode=Upper Bit Location + Width  bit1=5  base1=LSB of Input  bit0=0  base0=LSB of Input  XmcBlockStatus=1  maskContainerNames=group1  block_type=slice  block_config=sysgen:Slice_config
  Slice6 : hdlBasic/Slice  nbits=1  boolean_output=on  mode=Upper Bit Location + Width  bit1=6  base1=LSB of Input  bit0=0  base0=LSB of Input  XmcBlockStatus=1  maskContainerNames=group1  block_type=slice  block_config=sysgen:Slice_config
  Slice7 : hdlBasic/Slice  nbits=1  boolean_output=on  mode=Upper Bit Location + Width  bit1=7  base1=LSB of Input  bit0=0  base0=LSB of Input  XmcBlockStatus=1  maskContainerNames=group1  block_type=slice  block_config=sysgen:Slice_config
  OddParity : Outport
  wires:
  Logical/1 -> Logical2/1
  Slice3/1 -> Logical3/1
  Slice1/1 -> Logical4/1
  Logical2/1 -> Logical6/1
  Logical1/1 -> Logical2/2
  Slice/1 -> Logical4/2
  Slice4/1 -> Logical1/2
  Slice5/1 -> Logical1/1
  Logical4/1 -> Logical5/2
  Logical3/1 -> Logical5/1
  Slice7/1 -> Logical/1
  Slice6/1 -> Logical/2
  Slice2/1 -> Logical3/2
  Logical5/1 -> Logical6/2
  Data In/1 -> Slice7/1, Slice6/1, Slice5/1, Slice/1, Slice1/1, Slice2/1, Slice3/1, Slice4/1
  Logical6/1 -> OddParity/1
